simulink model "HANcoder_E407_TTA_Template_DS_V6"  (R2023a)
settings: Solver=FixedStepDiscrete  StartTime=0.0  StopTime=1  FixedStep=0.01  RelTol=1e-3
PreLoadFcn:
  | librarySetup
  | eval([bdroot,'_startup']) %Calling [modelName]_startup.m
values from neighbouring files (symbols this model uses):
  basic_cycle_duration_bc0 = TM_Reset_Board   + COMP_duration    (= 372)    [HANcoder_E407_TTA_Template_DS_V1_startup.m]    (also in HANcoder_E407_TTA_Template_DS_V2_startup.m; HANcoder_E407_TTA_Template_DS_V52_startup.m; HANcoder_E407_TTA_Template_DS_V5_startup.m; HANcoder_E407_TTA_Template_DS_V6_startup.m = 532)
  basic_cycle_duration_bc1 = basic_cycle_duration_bc0    (= 372)    [HANcoder_E407_TTA_Template_DS_V1_startup.m]    (also in HANcoder_E407_TTA_Template_DS_V2_startup.m; HANcoder_E407_TTA_Template_DS_V52_startup.m; HANcoder_E407_TTA_Template_DS_V5_startup.m; HANcoder_E407_TTA_Template_DS_V6_startup.m = 532)
  basic_cycle_duration_bc2 = basic_cycle_duration_bc0    (= 372)    [HANcoder_E407_TTA_Template_DS_V1_startup.m]    (also in HANcoder_E407_TTA_Template_DS_V2_startup.m; HANcoder_E407_TTA_Template_DS_V52_startup.m; HANcoder_E407_TTA_Template_DS_V5_startup.m; HANcoder_E407_TTA_Template_DS_V6_startup.m = 532)
  comm_delay_estimation1 = round(comm_delay_measured1*hardware_granularity/frequency_IRQ)    [HANcoder_E407_TTA_Template_DS_V1_startup.m]    (also in HANcoder_E407_TTA_Template_DS_V2_startup.m; HANcoder_E407_TTA_Template_DS_V52_startup.m; HANcoder_E407_TTA_Template_DS_V5_startup.m; HANcoder_E407_TTA_Template_DS_V6_startup.m)
  comm_delay_estimation2 = round(comm_delay_measured2*hardware_granularity/frequency_IRQ)    [HANcoder_E407_TTA_Template_DS_V1_startup.m]    (also in HANcoder_E407_TTA_Template_DS_V2_startup.m; HANcoder_E407_TTA_Template_DS_V52_startup.m; HANcoder_E407_TTA_Template_DS_V5_startup.m; HANcoder_E407_TTA_Template_DS_V6_startup.m)
  COMM_Period = 80    [HANcoder_E407_TTA_Template_DS_V1_startup.m]    (also in HANcoder_E407_TTA_Template_DS_V2_startup.m; HANcoder_E407_TTA_Template_DS_V52_startup.m; HANcoder_E407_TTA_Template_DS_V5_startup.m; HANcoder_E407_TTA_Template_DS_V6_startup.m = 120)
  COMM_Phase1 = Simulink.Parameter    [HANcoder_E407_TTA_Template_DS_V1_startup.m]    (also in HANcoder_E407_TTA_Template_DS_V2_startup.m; HANcoder_E407_TTA_Template_DS_V52_startup.m; HANcoder_E407_TTA_Template_DS_V5_startup.m; HANcoder_E407_TTA_Template_DS_V6_startup.m)
  COMM_Phase2 = Simulink.Parameter    [HANcoder_E407_TTA_Template_DS_V1_startup.m]    (also in HANcoder_E407_TTA_Template_DS_V2_startup.m; HANcoder_E407_TTA_Template_DS_V52_startup.m; HANcoder_E407_TTA_Template_DS_V5_startup.m; HANcoder_E407_TTA_Template_DS_V6_startup.m)
  COMM_Phase_init1 = Simulink.Parameter    [HANcoder_E407_TTA_Template_DS_V1_startup.m]    (also in HANcoder_E407_TTA_Template_DS_V2_startup.m; HANcoder_E407_TTA_Template_DS_V52_startup.m; HANcoder_E407_TTA_Template_DS_V5_startup.m; HANcoder_E407_TTA_Template_DS_V6_startup.m)
  COMM_Phase_init2 = Simulink.Parameter    [HANcoder_E407_TTA_Template_DS_V1_startup.m]    (also in HANcoder_E407_TTA_Template_DS_V2_startup.m; HANcoder_E407_TTA_Template_DS_V52_startup.m; HANcoder_E407_TTA_Template_DS_V5_startup.m; HANcoder_E407_TTA_Template_DS_V6_startup.m)
  COMP_duration = 4    [HANcoder_E407_TTA_Template_DS_V1_startup.m]    (also in HANcoder_E407_TTA_Template_DS_V2_startup.m; HANcoder_E407_TTA_Template_DS_V52_startup.m; HANcoder_E407_TTA_Template_DS_V5_startup.m; HANcoder_E407_TTA_Template_DS_V6_startup.m)
  frequency_IRQ = 100    [HANcoder_E407_TTA_Template_DS_V1_startup.m]    (also in HANcoder_E407_TTA_Template_DS_V2_startup.m; HANcoder_E407_TTA_Template_DS_V52_startup.m; HANcoder_E407_TTA_Template_DS_V5_startup.m; HANcoder_E407_TTA_Template_DS_V6_startup.m)
  idle_time_init = basic_cycle_duration_bc0 + basic_cycle_duration_bc1    (= 744)    [HANcoder_E407_TTA_Template_DS_V1_startup.m]    (also in HANcoder_E407_TTA_Template_DS_V2_startup.m; HANcoder_E407_TTA_Template_DS_V52_startup.m = 1116; HANcoder_E407_TTA_Template_DS_V5_startup.m = 1116; HANcoder_E407_TTA_Template_DS_V6_startup.m = 1596)
  L0b = 0.5    [HANcoder_E407_TTA_Template_DS_V52_startup.m]    (also in HANcoder_E407_TTA_Template_DS_V5_startup.m; HANcoder_E407_TTA_Template_DS_V6_startup.m)
  L0f = 5    [HANcoder_E407_TTA_Template_DS_V52_startup.m]    (also in HANcoder_E407_TTA_Template_DS_V5_startup.m; HANcoder_E407_TTA_Template_DS_V6_startup.m)
  L1f = 6    [HANcoder_E407_TTA_Template_DS_V52_startup.m]    (also in HANcoder_E407_TTA_Template_DS_V5_startup.m; HANcoder_E407_TTA_Template_DS_V6_startup.m)
  LA_Clock_Gr = 1    [HANcoder_E407_TTA_Template_DS_V1_startup.m]    (also in HANcoder_E407_TTA_Template_DS_V2_startup.m; HANcoder_E407_TTA_Template_DS_V52_startup.m; HANcoder_E407_TTA_Template_DS_V5_startup.m; HANcoder_E407_TTA_Template_DS_V6_startup.m)
  LA_COMM_dly = 1    [HANcoder_E407_TTA_Template_DS_V1_startup.m]    (also in HANcoder_E407_TTA_Template_DS_V2_startup.m; HANcoder_E407_TTA_Template_DS_V52_startup.m; HANcoder_E407_TTA_Template_DS_V5_startup.m; HANcoder_E407_TTA_Template_DS_V6_startup.m)
  LA_COMM_Err = 1    [HANcoder_E407_TTA_Template_DS_V1_startup.m]    (also in HANcoder_E407_TTA_Template_DS_V2_startup.m; HANcoder_E407_TTA_Template_DS_V52_startup.m; HANcoder_E407_TTA_Template_DS_V5_startup.m; HANcoder_E407_TTA_Template_DS_V6_startup.m)
  LA_E_Desync = 1    [HANcoder_E407_TTA_Template_DS_V1_startup.m]    (also in HANcoder_E407_TTA_Template_DS_V2_startup.m; HANcoder_E407_TTA_Template_DS_V52_startup.m; HANcoder_E407_TTA_Template_DS_V5_startup.m; HANcoder_E407_TTA_Template_DS_V6_startup.m)
  LA_MEX_Flag = 1    [HANcoder_E407_TTA_Template_DS_V1_startup.m]    (also in HANcoder_E407_TTA_Template_DS_V2_startup.m; HANcoder_E407_TTA_Template_DS_V52_startup.m; HANcoder_E407_TTA_Template_DS_V5_startup.m; HANcoder_E407_TTA_Template_DS_V6_startup.m)
  LA_Task_Act = 1    [HANcoder_E407_TTA_Template_DS_V1_startup.m]    (also in HANcoder_E407_TTA_Template_DS_V2_startup.m; HANcoder_E407_TTA_Template_DS_V52_startup.m; HANcoder_E407_TTA_Template_DS_V5_startup.m; HANcoder_E407_TTA_Template_DS_V6_startup.m)
  Master_Role = 1    [HANcoder_E407_TTA_Template_DS_V1_startup.m]    (also in HANcoder_E407_TTA_Template_DS_V2_startup.m; HANcoder_E407_TTA_Template_DS_V52_startup.m; HANcoder_E407_TTA_Template_DS_V5_startup.m; HANcoder_E407_TTA_Template_DS_V6_startup.m)
  matrix_rows = 3    [HANcoder_E407_TTA_Template_DS_V1_startup.m]    (also in HANcoder_E407_TTA_Template_DS_V2_startup.m; HANcoder_E407_TTA_Template_DS_V52_startup.m; HANcoder_E407_TTA_Template_DS_V5_startup.m; HANcoder_E407_TTA_Template_DS_V6_startup.m)
  max_desync = 15    [HANcoder_E407_TTA_Template_DS_V1_startup.m]    (also in HANcoder_E407_TTA_Template_DS_V2_startup.m; HANcoder_E407_TTA_Template_DS_V52_startup.m; HANcoder_E407_TTA_Template_DS_V5_startup.m; HANcoder_E407_TTA_Template_DS_V6_startup.m)
  max_num_msgs_CAN1 = 2^Tx_bit_number-1    (= 7)    [HANcoder_E407_TTA_Template_DS_V1_startup.m]    (also in HANcoder_E407_TTA_Template_DS_V2_startup.m; HANcoder_E407_TTA_Template_DS_V52_startup.m; HANcoder_E407_TTA_Template_DS_V5_startup.m; HANcoder_E407_TTA_Template_DS_V6_startup.m)
  max_num_msgs_CAN2 = max_num_msgs_CAN1    (= 7)    [HANcoder_E407_TTA_Template_DS_V1_startup.m]    (also in HANcoder_E407_TTA_Template_DS_V2_startup.m; HANcoder_E407_TTA_Template_DS_V52_startup.m; HANcoder_E407_TTA_Template_DS_V5_startup.m; HANcoder_E407_TTA_Template_DS_V6_startup.m)
  min_desync = (-1)*max_desync    (= -15)    [HANcoder_E407_TTA_Template_DS_V1_startup.m]    (also in HANcoder_E407_TTA_Template_DS_V2_startup.m; HANcoder_E407_TTA_Template_DS_V52_startup.m; HANcoder_E407_TTA_Template_DS_V5_startup.m; HANcoder_E407_TTA_Template_DS_V6_startup.m)
  PID_derivative = Simulink.Parameter    [HANcoder_E407_TTA_Template_DS_V52_startup.m]    (also in HANcoder_E407_TTA_Template_DS_V6_startup.m)
  PID_gain = Simulink.Parameter    [HANcoder_E407_TTA_Template_DS_V52_startup.m]    (also in HANcoder_E407_TTA_Template_DS_V6_startup.m)
  PID_integrator = Simulink.Parameter    [HANcoder_E407_TTA_Template_DS_V52_startup.m]    (also in HANcoder_E407_TTA_Template_DS_V6_startup.m)
  PotValue1_ID = 22    [HANcoder_E407_TTA_Template_DS_V1_startup.m]    (also in HANcoder_E407_TTA_Template_DS_V2_startup.m; HANcoder_E407_TTA_Template_DS_V52_startup.m; HANcoder_E407_TTA_Template_DS_V5_startup.m; HANcoder_E407_TTA_Template_DS_V6_startup.m)
  PotValue2_ID = 23    [HANcoder_E407_TTA_Template_DS_V1_startup.m]    (also in HANcoder_E407_TTA_Template_DS_V2_startup.m; HANcoder_E407_TTA_Template_DS_V52_startup.m; HANcoder_E407_TTA_Template_DS_V5_startup.m; HANcoder_E407_TTA_Template_DS_V6_startup.m)
  PotValue3_ID = 24    [HANcoder_E407_TTA_Template_DS_V1_startup.m]    (also in HANcoder_E407_TTA_Template_DS_V2_startup.m; HANcoder_E407_TTA_Template_DS_V52_startup.m; HANcoder_E407_TTA_Template_DS_V5_startup.m; HANcoder_E407_TTA_Template_DS_V6_startup.m)
  script_run = Simulink.Parameter    [HANcoder_E407_TTA_Template_DS_V1_startup.m]    (also in HANcoder_E407_TTA_Template_DS_V2_startup.m; HANcoder_E407_TTA_Template_DS_V52_startup.m; HANcoder_E407_TTA_Template_DS_V5_startup.m; HANcoder_E407_TTA_Template_DS_V6_startup.m)
  Slave_Role = 2    [HANcoder_E407_TTA_Template_DS_V1_startup.m]    (also in HANcoder_E407_TTA_Template_DS_V2_startup.m; HANcoder_E407_TTA_Template_DS_V52_startup.m; HANcoder_E407_TTA_Template_DS_V5_startup.m; HANcoder_E407_TTA_Template_DS_V6_startup.m)
  Sync_ID = 1    [HANcoder_E407_TTA_Template_DS_V1_startup.m]    (also in HANcoder_E407_TTA_Template_DS_V2_startup.m; HANcoder_E407_TTA_Template_DS_V52_startup.m; HANcoder_E407_TTA_Template_DS_V5_startup.m; HANcoder_E407_TTA_Template_DS_V6_startup.m)
  TM_Check_PotValue1 = TM_COMM_PotValue1 + COMM_duration    (= 174)    [HANcoder_E407_TTA_Template_DS_V1_startup.m]    (also in HANcoder_E407_TTA_Template_DS_V2_startup.m; HANcoder_E407_TTA_Template_DS_V52_startup.m; HANcoder_E407_TTA_Template_DS_V5_startup.m; HANcoder_E407_TTA_Template_DS_V6_startup.m = 254)
  TM_Check_PotValue2 = TM_COMM_PotValue2 + COMM_duration    (= 258)    [HANcoder_E407_TTA_Template_DS_V1_startup.m]    (also in HANcoder_E407_TTA_Template_DS_V2_startup.m; HANcoder_E407_TTA_Template_DS_V52_startup.m; HANcoder_E407_TTA_Template_DS_V5_startup.m; HANcoder_E407_TTA_Template_DS_V6_startup.m = 378)
  TM_Check_PotValue3 = TM_COMM_PotValue3 + COMM_duration    (= 342)    [HANcoder_E407_TTA_Template_DS_V1_startup.m]    (also in HANcoder_E407_TTA_Template_DS_V2_startup.m; HANcoder_E407_TTA_Template_DS_V52_startup.m; HANcoder_E407_TTA_Template_DS_V5_startup.m; HANcoder_E407_TTA_Template_DS_V6_startup.m = 502)
  TM_Check_Sync = TM_COMM_Sync   + COMM_duration    (= 80)    [HANcoder_E407_TTA_Template_DS_V1_startup.m]    (also in HANcoder_E407_TTA_Template_DS_V2_startup.m; HANcoder_E407_TTA_Template_DS_V52_startup.m; HANcoder_E407_TTA_Template_DS_V5_startup.m; HANcoder_E407_TTA_Template_DS_V6_startup.m = 120)
  TM_Check_TOuts = TM_Count_Vote3 + COMP_duration    (= 356)    [HANcoder_E407_TTA_Template_DS_V1_startup.m]    (also in HANcoder_E407_TTA_Template_DS_V2_startup.m; HANcoder_E407_TTA_Template_DS_V52_startup.m; HANcoder_E407_TTA_Template_DS_V5_startup.m; HANcoder_E407_TTA_Template_DS_V6_startup.m = 516)
  TM_Check_Trailer1Articulation = TM_COMM_Trailer1Articulation + COMM_duration    (= 170)    [HANcoder_E407_TTA_Template_DS_V1_startup.m]    (also in HANcoder_E407_TTA_Template_DS_V2_startup.m; HANcoder_E407_TTA_Template_DS_V52_startup.m; HANcoder_E407_TTA_Template_DS_V5_startup.m; HANcoder_E407_TTA_Template_DS_V6_startup.m = 250)
  TM_Check_Trailer2Articulation = TM_COMM_Trailer2Articulation + COMM_duration    (= 254)    [HANcoder_E407_TTA_Template_DS_V1_startup.m]    (also in HANcoder_E407_TTA_Template_DS_V2_startup.m; HANcoder_E407_TTA_Template_DS_V52_startup.m; HANcoder_E407_TTA_Template_DS_V5_startup.m; HANcoder_E407_TTA_Template_DS_V6_startup.m = 374)
  TM_Check_Vote1 = TM_COMM_Vote1  + COMM_duration    (= 172)    [HANcoder_E407_TTA_Template_DS_V1_startup.m]    (also in HANcoder_E407_TTA_Template_DS_V2_startup.m; HANcoder_E407_TTA_Template_DS_V52_startup.m; HANcoder_E407_TTA_Template_DS_V5_startup.m; HANcoder_E407_TTA_Template_DS_V6_startup.m = 252)
  TM_Check_Vote2 = TM_COMM_Vote2  + COMM_duration    (= 260)    [HANcoder_E407_TTA_Template_DS_V1_startup.m]    (also in HANcoder_E407_TTA_Template_DS_V2_startup.m; HANcoder_E407_TTA_Template_DS_V52_startup.m; HANcoder_E407_TTA_Template_DS_V5_startup.m; HANcoder_E407_TTA_Template_DS_V6_startup.m = 380)
  TM_Check_Vote3 = TM_COMM_Vote3  + COMM_duration    (= 348)    [HANcoder_E407_TTA_Template_DS_V1_startup.m]    (also in HANcoder_E407_TTA_Template_DS_V2_startup.m; HANcoder_E407_TTA_Template_DS_V52_startup.m; HANcoder_E407_TTA_Template_DS_V5_startup.m; HANcoder_E407_TTA_Template_DS_V6_startup.m = 508)
  TM_COMM_PotValue1 = TM_ReadPot + COMP_duration    (= 94)    [HANcoder_E407_TTA_Template_DS_V1_startup.m]    (also in HANcoder_E407_TTA_Template_DS_V2_startup.m; HANcoder_E407_TTA_Template_DS_V52_startup.m; HANcoder_E407_TTA_Template_DS_V5_startup.m; HANcoder_E407_TTA_Template_DS_V6_startup.m = 134)
  TM_COMM_PotValue2 = TM_Check_PotValue1 + COMP_duration    (= 178)    [HANcoder_E407_TTA_Template_DS_V1_startup.m]    (also in HANcoder_E407_TTA_Template_DS_V2_startup.m; HANcoder_E407_TTA_Template_DS_V52_startup.m; HANcoder_E407_TTA_Template_DS_V5_startup.m; HANcoder_E407_TTA_Template_DS_V6_startup.m = 258)
  TM_COMM_PotValue3 = TM_Check_PotValue2 + COMP_duration    (= 262)    [HANcoder_E407_TTA_Template_DS_V1_startup.m]    (also in HANcoder_E407_TTA_Template_DS_V2_startup.m; HANcoder_E407_TTA_Template_DS_V52_startup.m; HANcoder_E407_TTA_Template_DS_V5_startup.m; HANcoder_E407_TTA_Template_DS_V6_startup.m = 382)
  TM_COMM_Sync = basic_cycle_start    (= 0)    [HANcoder_E407_TTA_Template_DS_V1_startup.m]    (also in HANcoder_E407_TTA_Template_DS_V2_startup.m; HANcoder_E407_TTA_Template_DS_V52_startup.m; HANcoder_E407_TTA_Template_DS_V5_startup.m; HANcoder_E407_TTA_Template_DS_V6_startup.m)
  TM_COMM_Trailer1Articulation = TM_Update_LT_2 + COMP_duration    (= 90)    [HANcoder_E407_TTA_Template_DS_V1_startup.m]    (also in HANcoder_E407_TTA_Template_DS_V2_startup.m; HANcoder_E407_TTA_Template_DS_V52_startup.m; HANcoder_E407_TTA_Template_DS_V5_startup.m; HANcoder_E407_TTA_Template_DS_V6_startup.m = 130)
  TM_COMM_Trailer2Articulation = TM_Check_Trailer1Articulation + COMP_duration    (= 174)    [HANcoder_E407_TTA_Template_DS_V1_startup.m]    (also in HANcoder_E407_TTA_Template_DS_V2_startup.m; HANcoder_E407_TTA_Template_DS_V52_startup.m; HANcoder_E407_TTA_Template_DS_V5_startup.m; HANcoder_E407_TTA_Template_DS_V6_startup.m = 254)
  TM_COMM_Vote1 = TM_Vote_Dec    + COMP_duration    (= 92)    [HANcoder_E407_TTA_Template_DS_V1_startup.m]    (also in HANcoder_E407_TTA_Template_DS_V2_startup.m; HANcoder_E407_TTA_Template_DS_V52_startup.m; HANcoder_E407_TTA_Template_DS_V5_startup.m; HANcoder_E407_TTA_Template_DS_V6_startup.m = 132)
  TM_COMM_Vote2 = TM_Count_Vote1 + COMP_duration    (= 180)    [HANcoder_E407_TTA_Template_DS_V1_startup.m]    (also in HANcoder_E407_TTA_Template_DS_V2_startup.m; HANcoder_E407_TTA_Template_DS_V52_startup.m; HANcoder_E407_TTA_Template_DS_V5_startup.m; HANcoder_E407_TTA_Template_DS_V6_startup.m = 260)
  TM_COMM_Vote3 = TM_Count_Vote2 + COMP_duration    (= 268)    [HANcoder_E407_TTA_Template_DS_V1_startup.m]    (also in HANcoder_E407_TTA_Template_DS_V2_startup.m; HANcoder_E407_TTA_Template_DS_V52_startup.m; HANcoder_E407_TTA_Template_DS_V5_startup.m; HANcoder_E407_TTA_Template_DS_V6_startup.m = 388)
  TM_Count_Vote1 = TM_Check_Vote1 + COMP_duration    (= 176)    [HANcoder_E407_TTA_Template_DS_V1_startup.m]    (also in HANcoder_E407_TTA_Template_DS_V2_startup.m; HANcoder_E407_TTA_Template_DS_V52_startup.m; HANcoder_E407_TTA_Template_DS_V5_startup.m; HANcoder_E407_TTA_Template_DS_V6_startup.m = 256)
  TM_Count_Vote2 = TM_Check_Vote2 + COMP_duration    (= 264)    [HANcoder_E407_TTA_Template_DS_V1_startup.m]    (also in HANcoder_E407_TTA_Template_DS_V2_startup.m; HANcoder_E407_TTA_Template_DS_V52_startup.m; HANcoder_E407_TTA_Template_DS_V5_startup.m; HANcoder_E407_TTA_Template_DS_V6_startup.m = 384)
  TM_Count_Vote3 = TM_Check_Vote3 + COMP_duration    (= 352)    [HANcoder_E407_TTA_Template_DS_V1_startup.m]    (also in HANcoder_E407_TTA_Template_DS_V2_startup.m; HANcoder_E407_TTA_Template_DS_V52_startup.m; HANcoder_E407_TTA_Template_DS_V5_startup.m; HANcoder_E407_TTA_Template_DS_V6_startup.m = 512)
  TM_Data_bc0 = TM_COMM_Sync    (= 0)    [HANcoder_E407_TTA_Template_DS_V1_startup.m]    (also in HANcoder_E407_TTA_Template_DS_V2_startup.m; HANcoder_E407_TTA_Template_DS_V52_startup.m; HANcoder_E407_TTA_Template_DS_V5_startup.m; HANcoder_E407_TTA_Template_DS_V6_startup.m)
  TM_Data_bc1 = TM_Data_bc0(1:4)    [HANcoder_E407_TTA_Template_DS_V1_startup.m]    (also in HANcoder_E407_TTA_Template_DS_V2_startup.m; HANcoder_E407_TTA_Template_DS_V52_startup.m; HANcoder_E407_TTA_Template_DS_V5_startup.m; HANcoder_E407_TTA_Template_DS_V6_startup.m)
  TM_Data_bc2 = TM_Data_bc0(1:4)    [HANcoder_E407_TTA_Template_DS_V1_startup.m]    (also in HANcoder_E407_TTA_Template_DS_V2_startup.m; HANcoder_E407_TTA_Template_DS_V52_startup.m; HANcoder_E407_TTA_Template_DS_V5_startup.m; HANcoder_E407_TTA_Template_DS_V6_startup.m)
  TM_InverseKinematics = TM_Check_Trailer2Articulation + COMP_duration    (= 258)    [HANcoder_E407_TTA_Template_DS_V1_startup.m]    (also in HANcoder_E407_TTA_Template_DS_V2_startup.m; HANcoder_E407_TTA_Template_DS_V52_startup.m; HANcoder_E407_TTA_Template_DS_V5_startup.m; HANcoder_E407_TTA_Template_DS_V6_startup.m = 378)
  TM_New_Master = TM_Check_TOuts + COMP_duration    (= 360)    [HANcoder_E407_TTA_Template_DS_V1_startup.m]    (also in HANcoder_E407_TTA_Template_DS_V2_startup.m; HANcoder_E407_TTA_Template_DS_V52_startup.m; HANcoder_E407_TTA_Template_DS_V5_startup.m; HANcoder_E407_TTA_Template_DS_V6_startup.m = 520)
  TM_PotVote = TM_COMM_PotValue3 + COMP_duration    (= 266)    [HANcoder_E407_TTA_Template_DS_V1_startup.m]    (also in HANcoder_E407_TTA_Template_DS_V2_startup.m; HANcoder_E407_TTA_Template_DS_V52_startup.m; HANcoder_E407_TTA_Template_DS_V5_startup.m; HANcoder_E407_TTA_Template_DS_V6_startup.m = 386)
  TM_ReadPot = TM_Update_LT_2 + COMP_duration    (= 90)    [HANcoder_E407_TTA_Template_DS_V1_startup.m]    (also in HANcoder_E407_TTA_Template_DS_V2_startup.m; HANcoder_E407_TTA_Template_DS_V52_startup.m; HANcoder_E407_TTA_Template_DS_V5_startup.m; HANcoder_E407_TTA_Template_DS_V6_startup.m = 130)
  TM_Reset_Board = TM_Reset_Var   + COMP_duration    (= 368)    [HANcoder_E407_TTA_Template_DS_V1_startup.m]    (also in HANcoder_E407_TTA_Template_DS_V2_startup.m; HANcoder_E407_TTA_Template_DS_V52_startup.m; HANcoder_E407_TTA_Template_DS_V5_startup.m; HANcoder_E407_TTA_Template_DS_V6_startup.m = 528)
  TM_Reset_Var = TM_New_Master  + COMP_duration    (= 364)    [HANcoder_E407_TTA_Template_DS_V1_startup.m]    (also in HANcoder_E407_TTA_Template_DS_V2_startup.m; HANcoder_E407_TTA_Template_DS_V52_startup.m; HANcoder_E407_TTA_Template_DS_V5_startup.m; HANcoder_E407_TTA_Template_DS_V6_startup.m = 524)
  TM_Reset_Var_bc1 = TM_Data_bc1(end) + COMP_duration    [HANcoder_E407_TTA_Template_DS_V1_startup.m]    (also in HANcoder_E407_TTA_Template_DS_V2_startup.m; HANcoder_E407_TTA_Template_DS_V52_startup.m; HANcoder_E407_TTA_Template_DS_V5_startup.m; HANcoder_E407_TTA_Template_DS_V6_startup.m)
  TM_Reset_Var_bc1_2 = TM_Reset_Var_bc1 +2    [HANcoder_E407_TTA_Template_DS_V1_startup.m]    (also in HANcoder_E407_TTA_Template_DS_V2_startup.m; HANcoder_E407_TTA_Template_DS_V52_startup.m; HANcoder_E407_TTA_Template_DS_V5_startup.m; HANcoder_E407_TTA_Template_DS_V6_startup.m)
  TM_Reset_Var_bc2 = TM_Data_bc2(end) + COMP_duration    [HANcoder_E407_TTA_Template_DS_V1_startup.m]    (also in HANcoder_E407_TTA_Template_DS_V2_startup.m; HANcoder_E407_TTA_Template_DS_V52_startup.m; HANcoder_E407_TTA_Template_DS_V5_startup.m; HANcoder_E407_TTA_Template_DS_V6_startup.m)
  TM_Reset_Var_bc2_2 = TM_Reset_Var_bc2 +2    [HANcoder_E407_TTA_Template_DS_V1_startup.m]    (also in HANcoder_E407_TTA_Template_DS_V2_startup.m; HANcoder_E407_TTA_Template_DS_V52_startup.m; HANcoder_E407_TTA_Template_DS_V5_startup.m; HANcoder_E407_TTA_Template_DS_V6_startup.m)
  TM_Type_bc0 = COMM    (= 0)    [HANcoder_E407_TTA_Template_DS_V1_startup.m]    (also in HANcoder_E407_TTA_Template_DS_V2_startup.m; HANcoder_E407_TTA_Template_DS_V52_startup.m; HANcoder_E407_TTA_Template_DS_V5_startup.m; HANcoder_E407_TTA_Template_DS_V6_startup.m)
  TM_Type_bc1 = TM_Type_bc0(1:4)    [HANcoder_E407_TTA_Template_DS_V1_startup.m]    (also in HANcoder_E407_TTA_Template_DS_V2_startup.m; HANcoder_E407_TTA_Template_DS_V52_startup.m; HANcoder_E407_TTA_Template_DS_V5_startup.m; HANcoder_E407_TTA_Template_DS_V6_startup.m)
  TM_Type_bc2 = TM_Type_bc0(1:4)    [HANcoder_E407_TTA_Template_DS_V1_startup.m]    (also in HANcoder_E407_TTA_Template_DS_V2_startup.m; HANcoder_E407_TTA_Template_DS_V52_startup.m; HANcoder_E407_TTA_Template_DS_V5_startup.m; HANcoder_E407_TTA_Template_DS_V6_startup.m)
  TM_Update_LT = TM_Check_Sync  + COMP_duration    (= 84)    [HANcoder_E407_TTA_Template_DS_V1_startup.m]    (also in HANcoder_E407_TTA_Template_DS_V2_startup.m; HANcoder_E407_TTA_Template_DS_V52_startup.m; HANcoder_E407_TTA_Template_DS_V5_startup.m; HANcoder_E407_TTA_Template_DS_V6_startup.m = 124)
  TM_Update_LT_2 = TM_Update_LT   + 2    (= 86)    [HANcoder_E407_TTA_Template_DS_V1_startup.m]    (also in HANcoder_E407_TTA_Template_DS_V2_startup.m; HANcoder_E407_TTA_Template_DS_V52_startup.m; HANcoder_E407_TTA_Template_DS_V5_startup.m; HANcoder_E407_TTA_Template_DS_V6_startup.m = 126)
  TM_Vote_Dec = TM_Update_LT   + COMP_duration    (= 88)    [HANcoder_E407_TTA_Template_DS_V1_startup.m]    (also in HANcoder_E407_TTA_Template_DS_V2_startup.m; HANcoder_E407_TTA_Template_DS_V52_startup.m; HANcoder_E407_TTA_Template_DS_V5_startup.m; HANcoder_E407_TTA_Template_DS_V6_startup.m = 128)
  Tractor_Board1 = 11    [HANcoder_E407_TTA_Template_DS_V1_startup.m]    (also in HANcoder_E407_TTA_Template_DS_V2_startup.m = 1; HANcoder_E407_TTA_Template_DS_V52_startup.m = 1; HANcoder_E407_TTA_Template_DS_V5_startup.m = 1; HANcoder_E407_TTA_Template_DS_V6_startup.m = 1)
  Tractor_Board2 = 12    [HANcoder_E407_TTA_Template_DS_V1_startup.m]    (also in HANcoder_E407_TTA_Template_DS_V2_startup.m = 2; HANcoder_E407_TTA_Template_DS_V52_startup.m = 2; HANcoder_E407_TTA_Template_DS_V5_startup.m = 2; HANcoder_E407_TTA_Template_DS_V6_startup.m = 2)
  Tractor_Board3 = 13    [HANcoder_E407_TTA_Template_DS_V1_startup.m]    (also in HANcoder_E407_TTA_Template_DS_V2_startup.m = 3; HANcoder_E407_TTA_Template_DS_V52_startup.m = 3; HANcoder_E407_TTA_Template_DS_V5_startup.m = 3; HANcoder_E407_TTA_Template_DS_V6_startup.m = 3)
  Trailer1_Articulation_ID = 31    [HANcoder_E407_TTA_Template_DS_V1_startup.m]    (also in HANcoder_E407_TTA_Template_DS_V2_startup.m; HANcoder_E407_TTA_Template_DS_V52_startup.m; HANcoder_E407_TTA_Template_DS_V5_startup.m; HANcoder_E407_TTA_Template_DS_V6_startup.m)
  Trailer1_Board1 = 2    [HANcoder_E407_TTA_Template_DS_V1_startup.m]    (also in HANcoder_E407_TTA_Template_DS_V2_startup.m = 4; HANcoder_E407_TTA_Template_DS_V52_startup.m = 4; HANcoder_E407_TTA_Template_DS_V5_startup.m = 4; HANcoder_E407_TTA_Template_DS_V6_startup.m = 4)
  Trailer1_Board2 = 3    [HANcoder_E407_TTA_Template_DS_V1_startup.m]    (also in HANcoder_E407_TTA_Template_DS_V2_startup.m = 5; HANcoder_E407_TTA_Template_DS_V52_startup.m = 5; HANcoder_E407_TTA_Template_DS_V5_startup.m = 5; HANcoder_E407_TTA_Template_DS_V6_startup.m = 5)
  Trailer1_Board3 = 4    [HANcoder_E407_TTA_Template_DS_V1_startup.m]    (also in HANcoder_E407_TTA_Template_DS_V2_startup.m = 6; HANcoder_E407_TTA_Template_DS_V52_startup.m = 6; HANcoder_E407_TTA_Template_DS_V5_startup.m = 6; HANcoder_E407_TTA_Template_DS_V6_startup.m = 6)
  Trailer2_Articulation_ID = 32    [HANcoder_E407_TTA_Template_DS_V1_startup.m]    (also in HANcoder_E407_TTA_Template_DS_V2_startup.m; HANcoder_E407_TTA_Template_DS_V52_startup.m; HANcoder_E407_TTA_Template_DS_V5_startup.m; HANcoder_E407_TTA_Template_DS_V6_startup.m)
  Trailer2_Board1 = 5    [HANcoder_E407_TTA_Template_DS_V1_startup.m]    (also in HANcoder_E407_TTA_Template_DS_V2_startup.m = 7; HANcoder_E407_TTA_Template_DS_V52_startup.m = 7; HANcoder_E407_TTA_Template_DS_V5_startup.m = 7; HANcoder_E407_TTA_Template_DS_V6_startup.m = 7)
  Trailer2_Board2 = 6    [HANcoder_E407_TTA_Template_DS_V1_startup.m]    (also in HANcoder_E407_TTA_Template_DS_V2_startup.m = 8; HANcoder_E407_TTA_Template_DS_V52_startup.m = 8; HANcoder_E407_TTA_Template_DS_V5_startup.m = 8; HANcoder_E407_TTA_Template_DS_V6_startup.m = 8)
  Trailer2_Board3 = 7    [HANcoder_E407_TTA_Template_DS_V1_startup.m]    (also in HANcoder_E407_TTA_Template_DS_V2_startup.m = 9; HANcoder_E407_TTA_Template_DS_V52_startup.m = 9; HANcoder_E407_TTA_Template_DS_V5_startup.m = 9; HANcoder_E407_TTA_Template_DS_V6_startup.m = 9)
  V1 = -0.000000001    (= -1e-09)    [HANcoder_E407_TTA_Template_DS_V52_startup.m]    (also in HANcoder_E407_TTA_Template_DS_V5_startup.m; HANcoder_E407_TTA_Template_DS_V6_startup.m)
  V2 = -0.000000001    (= -1e-09)    [HANcoder_E407_TTA_Template_DS_V52_startup.m]    (also in HANcoder_E407_TTA_Template_DS_V5_startup.m; HANcoder_E407_TTA_Template_DS_V6_startup.m)
  Vote1_ID = 11    [HANcoder_E407_TTA_Template_DS_V1_startup.m]    (also in HANcoder_E407_TTA_Template_DS_V2_startup.m; HANcoder_E407_TTA_Template_DS_V52_startup.m; HANcoder_E407_TTA_Template_DS_V5_startup.m; HANcoder_E407_TTA_Template_DS_V6_startup.m)
  Vote2_ID = 12    [HANcoder_E407_TTA_Template_DS_V1_startup.m]    (also in HANcoder_E407_TTA_Template_DS_V2_startup.m; HANcoder_E407_TTA_Template_DS_V52_startup.m; HANcoder_E407_TTA_Template_DS_V5_startup.m; HANcoder_E407_TTA_Template_DS_V6_startup.m)
  Vote3_ID = 13    [HANcoder_E407_TTA_Template_DS_V1_startup.m]    (also in HANcoder_E407_TTA_Template_DS_V2_startup.m; HANcoder_E407_TTA_Template_DS_V52_startup.m; HANcoder_E407_TTA_Template_DS_V5_startup.m; HANcoder_E407_TTA_Template_DS_V6_startup.m)
undefined symbols (not defined in the file or in its folder): A0, A1, A2, A3, A4, A5, CON2, CON3, CON4, D10, D12, D13, D6, D7, D8, D9
libraries: hdlsllib x136, simulink x39, HANcoder_STM32_Target x31, simulink_extras x8, dspstat3 x2, slpidlib x1
(part 14 of 42)

== system HANcoder_E407_TTA_Template_DS_V6/HANcoder STM32 Target - E407-STM32 algorithm/TTA CAN System/CAN2 Recieve1/RxID_CAN/PotValue2_ID_CAN3/CAN receive1 ==
  In1 : Inport
  Enabled Subsystem : Subsystem  TreatAsAtomicUnit=on
  S-Function : M-S-Function  FunctionName=sfcn_can_receive  Parameters=tsamp, canBus, outputNumber, dataType, byteOrder
  Out1 : Outport  VectorParamsAs1DForOutWhenUnconnected=off
  Out2 : Outport  Port=2  VectorParamsAs1DForOutWhenUnconnected=off
  Out3 : Outport  Port=3  VectorParamsAs1DForOutWhenUnconnected=off
  Out4 : Outport  Port=4  VectorParamsAs1DForOutWhenUnconnected=off
  Out5 : Outport  Port=5  VectorParamsAs1DForOutWhenUnconnected=off
  Out6 : Outport  Port=6  VectorParamsAs1DForOutWhenUnconnected=off
  Out7 : Outport  Port=7  VectorParamsAs1DForOutWhenUnconnected=off
  Out8 : Outport  Port=8  VectorParamsAs1DForOutWhenUnconnected=off
  Out9 : Outport  Port=9  VectorParamsAs1DForOutWhenUnconnected=off
  wires:
  In1/1 -> S-Function/1
  S-Function/1 -> Enabled Subsystem/Enable, Out1/1
  S-Function/2 -> Enabled Subsystem/1(In1)
  S-Function/3 -> Enabled Subsystem/2(In2)
  Enabled Subsystem/1(Out1) -> Out2/1
  Enabled Subsystem/2(Out2) -> Out3/1
  Enabled Subsystem/3(Out3) -> Out4/1
  Enabled Subsystem/4(Out4) -> Out5/1
  Enabled Subsystem/5(Out5) -> Out6/1
  Enabled Subsystem/6(Out6) -> Out7/1
  Enabled Subsystem/7(Out7) -> Out8/1
  Enabled Subsystem/8(Out8) -> Out9/1
  S-Function/6 -> Enabled Subsystem/5(In5)
  S-Function/7 -> Enabled Subsystem/6(In6)
  S-Function/8 -> Enabled Subsystem/7(In7)
  S-Function/5 -> Enabled Subsystem/4(In4)
  S-Function/4 -> Enabled Subsystem/3(In3)
  S-Function/9 -> Enabled Subsystem/8(In8)

== system HANcoder_E407_TTA_Template_DS_V6/HANcoder STM32 Target - E407-STM32 algorithm/TTA CAN System/CAN2 Recieve1/RxID_CAN/PotValue2_ID_CAN4/CAN receive1 ==
  In1 : Inport
  Enabled Subsystem : Subsystem  TreatAsAtomicUnit=on
  S-Function : M-S-Function  FunctionName=sfcn_can_receive  Parameters=tsamp, canBus, outputNumber, dataType, byteOrder
  Out1 : Outport  VectorParamsAs1DForOutWhenUnconnected=off
  Out2 : Outport  Port=2  VectorParamsAs1DForOutWhenUnconnected=off
  Out3 : Outport  Port=3  VectorParamsAs1DForOutWhenUnconnected=off
  Out4 : Outport  Port=4  VectorParamsAs1DForOutWhenUnconnected=off
  Out5 : Outport  Port=5  VectorParamsAs1DForOutWhenUnconnected=off
  Out6 : Outport  Port=6  VectorParamsAs1DForOutWhenUnconnected=off
  Out7 : Outport  Port=7  VectorParamsAs1DForOutWhenUnconnected=off
  Out8 : Outport  Port=8  VectorParamsAs1DForOutWhenUnconnected=off
  Out9 : Outport  Port=9  VectorParamsAs1DForOutWhenUnconnected=off
  wires:
  In1/1 -> S-Function/1
  S-Function/1 -> Enabled Subsystem/Enable, Out1/1
  S-Function/2 -> Enabled Subsystem/1(In1)
  S-Function/3 -> Enabled Subsystem/2(In2)
  Enabled Subsystem/1(Out1) -> Out2/1
  Enabled Subsystem/2(Out2) -> Out3/1
  Enabled Subsystem/3(Out3) -> Out4/1
  Enabled Subsystem/4(Out4) -> Out5/1
  Enabled Subsystem/5(Out5) -> Out6/1
  Enabled Subsystem/6(Out6) -> Out7/1
  Enabled Subsystem/7(Out7) -> Out8/1
  Enabled Subsystem/8(Out8) -> Out9/1
  S-Function/6 -> Enabled Subsystem/5(In5)
  S-Function/7 -> Enabled Subsystem/6(In6)
  S-Function/8 -> Enabled Subsystem/7(In7)
  S-Function/5 -> Enabled Subsystem/4(In4)
  S-Function/4 -> Enabled Subsystem/3(In3)
  S-Function/9 -> Enabled Subsystem/8(In8)

== system HANcoder_E407_TTA_Template_DS_V6/HANcoder STM32 Target - E407-STM32 algorithm/TTA CAN System/CAN2 Recieve1/RxID_CAN/PotValue2_ID_CAN5/CAN receive1 ==
  In1 : Inport
  Enabled Subsystem : Subsystem  TreatAsAtomicUnit=on
  S-Function : M-S-Function  FunctionName=sfcn_can_receive  Parameters=tsamp, canBus, outputNumber, dataType, byteOrder
  Out1 : Outport  VectorParamsAs1DForOutWhenUnconnected=off
  Out2 : Outport  Port=2  VectorParamsAs1DForOutWhenUnconnected=off
  Out3 : Outport  Port=3  VectorParamsAs1DForOutWhenUnconnected=off
  Out4 : Outport  Port=4  VectorParamsAs1DForOutWhenUnconnected=off
  Out5 : Outport  Port=5  VectorParamsAs1DForOutWhenUnconnected=off
  Out6 : Outport  Port=6  VectorParamsAs1DForOutWhenUnconnected=off
  Out7 : Outport  Port=7  VectorParamsAs1DForOutWhenUnconnected=off
  Out8 : Outport  Port=8  VectorParamsAs1DForOutWhenUnconnected=off
  Out9 : Outport  Port=9  VectorParamsAs1DForOutWhenUnconnected=off
  wires:
  In1/1 -> S-Function/1
  S-Function/1 -> Enabled Subsystem/Enable, Out1/1
  S-Function/2 -> Enabled Subsystem/1(In1)
  S-Function/3 -> Enabled Subsystem/2(In2)
  Enabled Subsystem/1(Out1) -> Out2/1
  Enabled Subsystem/2(Out2) -> Out3/1
  Enabled Subsystem/3(Out3) -> Out4/1
  Enabled Subsystem/4(Out4) -> Out5/1
  Enabled Subsystem/5(Out5) -> Out6/1
  Enabled Subsystem/6(Out6) -> Out7/1
  Enabled Subsystem/7(Out7) -> Out8/1
  Enabled Subsystem/8(Out8) -> Out9/1
  S-Function/6 -> Enabled Subsystem/5(In5)
  S-Function/7 -> Enabled Subsystem/6(In6)
  S-Function/8 -> Enabled Subsystem/7(In7)
  S-Function/5 -> Enabled Subsystem/4(In4)
  S-Function/4 -> Enabled Subsystem/3(In3)
  S-Function/9 -> Enabled Subsystem/8(In8)

== system HANcoder_E407_TTA_Template_DS_V6/HANcoder STM32 Target - E407-STM32 algorithm/TTA CAN System/CAN2 Recieve1/RxID_CAN/PotValue2_ID_CAN6/CAN receive1 ==
  In1 : Inport
  Enabled Subsystem : Subsystem  TreatAsAtomicUnit=on
  S-Function : M-S-Function  FunctionName=sfcn_can_receive  Parameters=tsamp, canBus, outputNumber, dataType, byteOrder
  Out1 : Outport  VectorParamsAs1DForOutWhenUnconnected=off
  Out2 : Outport  Port=2  VectorParamsAs1DForOutWhenUnconnected=off
  Out3 : Outport  Port=3  VectorParamsAs1DForOutWhenUnconnected=off
  Out4 : Outport  Port=4  VectorParamsAs1DForOutWhenUnconnected=off
  Out5 : Outport  Port=5  VectorParamsAs1DForOutWhenUnconnected=off
  Out6 : Outport  Port=6  VectorParamsAs1DForOutWhenUnconnected=off
  Out7 : Outport  Port=7  VectorParamsAs1DForOutWhenUnconnected=off
  Out8 : Outport  Port=8  VectorParamsAs1DForOutWhenUnconnected=off
  Out9 : Outport  Port=9  VectorParamsAs1DForOutWhenUnconnected=off
  wires:
  In1/1 -> S-Function/1
  S-Function/1 -> Enabled Subsystem/Enable, Out1/1
  S-Function/2 -> Enabled Subsystem/1(In1)
  S-Function/3 -> Enabled Subsystem/2(In2)
  Enabled Subsystem/1(Out1) -> Out2/1
  Enabled Subsystem/2(Out2) -> Out3/1
  Enabled Subsystem/3(Out3) -> Out4/1
  Enabled Subsystem/4(Out4) -> Out5/1
  Enabled Subsystem/5(Out5) -> Out6/1
  Enabled Subsystem/6(Out6) -> Out7/1
  Enabled Subsystem/7(Out7) -> Out8/1
  Enabled Subsystem/8(Out8) -> Out9/1
  S-Function/6 -> Enabled Subsystem/5(In5)
  S-Function/7 -> Enabled Subsystem/6(In6)
  S-Function/8 -> Enabled Subsystem/7(In7)
  S-Function/5 -> Enabled Subsystem/4(In4)
  S-Function/4 -> Enabled Subsystem/3(In3)
  S-Function/9 -> Enabled Subsystem/8(In8)

== system HANcoder_E407_TTA_Template_DS_V6/HANcoder STM32 Target - E407-STM32 algorithm/TTA CAN System/CAN2 Recieve1/RxID_CAN/Sync_ID_CAN/CAN receive1 ==
  In1 : Inport
  Enabled Subsystem : Subsystem  TreatAsAtomicUnit=on
  S-Function : M-S-Function  FunctionName=sfcn_can_receive  Parameters=tsamp, canBus, outputNumber, dataType, byteOrder
  Out1 : Outport  VectorParamsAs1DForOutWhenUnconnected=off
  Out2 : Outport  Port=2  VectorParamsAs1DForOutWhenUnconnected=off
  Out3 : Outport  Port=3  VectorParamsAs1DForOutWhenUnconnected=off
  Out4 : Outport  Port=4  VectorParamsAs1DForOutWhenUnconnected=off
  Out5 : Outport  Port=5  VectorParamsAs1DForOutWhenUnconnected=off
  Out6 : Outport  Port=6  VectorParamsAs1DForOutWhenUnconnected=off
  Out7 : Outport  Port=7  VectorParamsAs1DForOutWhenUnconnected=off
  Out8 : Outport  Port=8  VectorParamsAs1DForOutWhenUnconnected=off
  Out9 : Outport  Port=9  VectorParamsAs1DForOutWhenUnconnected=off
  wires:
  S-Function/9 -> Enabled Subsystem/8(In8)
  S-Function/4 -> Enabled Subsystem/3(In3)
  S-Function/5 -> Enabled Subsystem/4(In4)
  S-Function/8 -> Enabled Subsystem/7(In7)
  S-Function/7 -> Enabled Subsystem/6(In6)
  S-Function/6 -> Enabled Subsystem/5(In5)
  Enabled Subsystem/8(Out8) -> Out9/1
  Enabled Subsystem/7(Out7) -> Out8/1
  Enabled Subsystem/6(Out6) -> Out7/1
  Enabled Subsystem/5(Out5) -> Out6/1
  Enabled Subsystem/4(Out4) -> Out5/1
  Enabled Subsystem/3(Out3) -> Out4/1
  Enabled Subsystem/2(Out2) -> Out3/1
  Enabled Subsystem/1(Out1) -> Out2/1
  S-Function/3 -> Enabled Subsystem/2(In2)
  S-Function/2 -> Enabled Subsystem/1(In1)
  S-Function/1 -> Out1/1, Enabled Subsystem/Enable
  In1/1 -> S-Function/1

== system HANcoder_E407_TTA_Template_DS_V6/HANcoder STM32 Target - E407-STM32 algorithm/TTA CAN System/CAN2 Recieve1/RxID_CAN/Vote1_ID_CAN/CAN receive1 ==
  In1 : Inport
  Enabled Subsystem : Subsystem  TreatAsAtomicUnit=on
  S-Function : M-S-Function  FunctionName=sfcn_can_receive  Parameters=tsamp, canBus, outputNumber, dataType, byteOrder
  Out1 : Outport  VectorParamsAs1DForOutWhenUnconnected=off
  Out2 : Outport  Port=2  VectorParamsAs1DForOutWhenUnconnected=off
  Out3 : Outport  Port=3  VectorParamsAs1DForOutWhenUnconnected=off
  Out4 : Outport  Port=4  VectorParamsAs1DForOutWhenUnconnected=off
  Out5 : Outport  Port=5  VectorParamsAs1DForOutWhenUnconnected=off
  Out6 : Outport  Port=6  VectorParamsAs1DForOutWhenUnconnected=off
  Out7 : Outport  Port=7  VectorParamsAs1DForOutWhenUnconnected=off
  Out8 : Outport  Port=8  VectorParamsAs1DForOutWhenUnconnected=off
  Out9 : Outport  Port=9  VectorParamsAs1DForOutWhenUnconnected=off
  wires:
  In1/1 -> S-Function/1
  S-Function/1 -> Enabled Subsystem/Enable, Out1/1
  S-Function/2 -> Enabled Subsystem/1(In1)
  S-Function/3 -> Enabled Subsystem/2(In2)
  Enabled Subsystem/1(Out1) -> Out2/1
  Enabled Subsystem/2(Out2) -> Out3/1
  Enabled Subsystem/3(Out3) -> Out4/1
  Enabled Subsystem/4(Out4) -> Out5/1
  Enabled Subsystem/5(Out5) -> Out6/1
  Enabled Subsystem/6(Out6) -> Out7/1
  Enabled Subsystem/7(Out7) -> Out8/1
  Enabled Subsystem/8(Out8) -> Out9/1
  S-Function/6 -> Enabled Subsystem/5(In5)
  S-Function/7 -> Enabled Subsystem/6(In6)
  S-Function/8 -> Enabled Subsystem/7(In7)
  S-Function/5 -> Enabled Subsystem/4(In4)
  S-Function/4 -> Enabled Subsystem/3(In3)
  S-Function/9 -> Enabled Subsystem/8(In8)

== system HANcoder_E407_TTA_Template_DS_V6/HANcoder STM32 Target - E407-STM32 algorithm/TTA CAN System/CAN2 Recieve1/RxID_CAN/Vote2_ID_CAN/CAN receive1 ==
  In1 : Inport
  Enabled Subsystem : Subsystem  TreatAsAtomicUnit=on
  S-Function : M-S-Function  FunctionName=sfcn_can_receive  Parameters=tsamp, canBus, outputNumber, dataType, byteOrder
  Out1 : Outport  VectorParamsAs1DForOutWhenUnconnected=off
  Out2 : Outport  Port=2  VectorParamsAs1DForOutWhenUnconnected=off
  Out3 : Outport  Port=3  VectorParamsAs1DForOutWhenUnconnected=off
  Out4 : Outport  Port=4  VectorParamsAs1DForOutWhenUnconnected=off
  Out5 : Outport  Port=5  VectorParamsAs1DForOutWhenUnconnected=off
  Out6 : Outport  Port=6  VectorParamsAs1DForOutWhenUnconnected=off
  Out7 : Outport  Port=7  VectorParamsAs1DForOutWhenUnconnected=off
  Out8 : Outport  Port=8  VectorParamsAs1DForOutWhenUnconnected=off
  Out9 : Outport  Port=9  VectorParamsAs1DForOutWhenUnconnected=off
  wires:
  In1/1 -> S-Function/1
  S-Function/1 -> Enabled Subsystem/Enable, Out1/1
  S-Function/2 -> Enabled Subsystem/1(In1)
  S-Function/3 -> Enabled Subsystem/2(In2)
  Enabled Subsystem/1(Out1) -> Out2/1
  Enabled Subsystem/2(Out2) -> Out3/1
  Enabled Subsystem/3(Out3) -> Out4/1
  Enabled Subsystem/4(Out4) -> Out5/1
  Enabled Subsystem/5(Out5) -> Out6/1
  Enabled Subsystem/6(Out6) -> Out7/1
  Enabled Subsystem/7(Out7) -> Out8/1
  Enabled Subsystem/8(Out8) -> Out9/1
  S-Function/6 -> Enabled Subsystem/5(In5)
  S-Function/7 -> Enabled Subsystem/6(In6)
  S-Function/8 -> Enabled Subsystem/7(In7)
  S-Function/5 -> Enabled Subsystem/4(In4)
  S-Function/4 -> Enabled Subsystem/3(In3)
  S-Function/9 -> Enabled Subsystem/8(In8)

== system HANcoder_E407_TTA_Template_DS_V6/HANcoder STM32 Target - E407-STM32 algorithm/TTA CAN System/CAN2 Recieve1/RxID_CAN/Vote3_ID_CAN/CAN receive1 ==
  In1 : Inport
  Enabled Subsystem : Subsystem  TreatAsAtomicUnit=on
  S-Function : M-S-Function  FunctionName=sfcn_can_receive  Parameters=tsamp, canBus, outputNumber, dataType, byteOrder
  Out1 : Outport  VectorParamsAs1DForOutWhenUnconnected=off
  Out2 : Outport  Port=2  VectorParamsAs1DForOutWhenUnconnected=off
  Out3 : Outport  Port=3  VectorParamsAs1DForOutWhenUnconnected=off
  Out4 : Outport  Port=4  VectorParamsAs1DForOutWhenUnconnected=off
  Out5 : Outport  Port=5  VectorParamsAs1DForOutWhenUnconnected=off
  Out6 : Outport  Port=6  VectorParamsAs1DForOutWhenUnconnected=off
  Out7 : Outport  Port=7  VectorParamsAs1DForOutWhenUnconnected=off
  Out8 : Outport  Port=8  VectorParamsAs1DForOutWhenUnconnected=off
  Out9 : Outport  Port=9  VectorParamsAs1DForOutWhenUnconnected=off
  wires:
  In1/1 -> S-Function/1
  S-Function/1 -> Enabled Subsystem/Enable, Out1/1
  S-Function/2 -> Enabled Subsystem/1(In1)
  S-Function/3 -> Enabled Subsystem/2(In2)
  Enabled Subsystem/1(Out1) -> Out2/1
  Enabled Subsystem/2(Out2) -> Out3/1
  Enabled Subsystem/3(Out3) -> Out4/1
  Enabled Subsystem/4(Out4) -> Out5/1
  Enabled Subsystem/5(Out5) -> Out6/1
  Enabled Subsystem/6(Out6) -> Out7/1
  Enabled Subsystem/7(Out7) -> Out8/1
  Enabled Subsystem/8(Out8) -> Out9/1
  S-Function/6 -> Enabled Subsystem/5(In5)
  S-Function/7 -> Enabled Subsystem/6(In6)
  S-Function/8 -> Enabled Subsystem/7(In7)
  S-Function/5 -> Enabled Subsystem/4(In4)
  S-Function/4 -> Enabled Subsystem/3(In3)
  S-Function/9 -> Enabled Subsystem/8(In8)

== system HANcoder_E407_TTA_Template_DS_V6/HANcoder STM32 Target - E407-STM32 algorithm/TTA CAN System/TTA System/Initialization/RoleID and Global Time init/Global Time Initialization Master ==
  note: Global Time Initialization
  Enable : EnablePort
  Board nr1 : Constant
  Cast : DataTypeConversion  OutDataTypeStr=uint16  SaturateOnIntegerOverflow=off  RndMeth=Floor
  Cast1 : DataTypeConversion  OutDataTypeStr=uint8  SaturateOnIntegerOverflow=off  RndMeth=Floor
  Data Store Write : DataStoreWrite  DataStoreName=Local_Ticks  IndexOptions=Index vector (dialog)  Indices=1  OutputSizes=1
  Data Store Write1 : DataStoreWrite  DataStoreName=basic_cycle_count  IndexOptions=Index vector (dialog)  Indices=1  OutputSizes=1
  Data Store Write3 : DataStoreWrite  DataStoreName=Master_ID  IndexOptions=Index vector (dialog)  Indices=1  OutputSizes=1
  Start : Constant  Value=0
  wires:
  Board nr1/1 -> Data Store Write3/1
  Start/1 -> Cast1/1, Cast/1
  Cast/1 -> Data Store Write/1
  Cast1/1 -> Data Store Write1/1

== system HANcoder_E407_TTA_Template_DS_V6/HANcoder STM32 Target - E407-STM32 algorithm/TTA CAN System/TTA System/Initialization/RoleID and Global Time init/Global Time Initialization Slave ==
  note: Sync has already been received, so we skip
      | the first comp tasks related to Update LT.
  note: Global Time Initialization
  note: Estimation of the Local Time when the message was sent
  Enable : EnablePort
  Bus Selector : BusSelector  OutputSignals=Buffer_1,Buffer_2,Buffer_3,Buffer_4,Buffer_5,Buffer_6,Buffer_7,Buffer_8
  Cast : DataTypeConversion  OutDataTypeStr=uint16  SaturateOnIntegerOverflow=off  RndMeth=Floor
  Cast1 : DataTypeConversion  OutDataTypeStr=double  SaturateOnIntegerOverflow=off  RndMeth=Floor
  Constant : Constant
  Constant1 : Constant  Value=COMM_Phase1
  Constant2 : Constant  Value=COMM_Phase2
  Constant3 : Constant  Value=TM_COMM_Sync
  Data Store Read : DataStoreRead  DataStoreName=New_Msg_Ready_CAN1  IndexOptions=Index vector (dialog)  Indices=1  OutputSizes=1
  Data Store Read1 : DataStoreRead  DataStoreName=Msg_Rx_CAN1  IndexOptions=Index vector (dialog)  Indices=1  OutputSizes=1
  Data Store Read2 : DataStoreRead  DataStoreName=Msg_Rx_CAN2  IndexOptions=Index vector (dialog)  Indices=1  OutputSizes=1
  Data Store Write1 : DataStoreWrite  DataStoreName=Local_Ticks  IndexOptions=Index vector (dialog)  Indices=1  OutputSizes=1
  Data Store Write2 : DataStoreWrite  DataStoreName=basic_cycle_count  IndexOptions=Index vector (dialog)  Indices=1  OutputSizes=1
  Data Store Write3 : DataStoreWrite  DataStoreName=Master_ID  IndexOptions=Index vector (dialog)  Indices=1  OutputSizes=1
  Data Store Write4 : DataStoreWrite  Priority=10  DataStoreName=BC0_Sync_processed  IndexOptions=Index vector (dialog)  Indices=1  OutputSizes=1
  Equal : RelationalOperator  Operator===  OutDataTypeStr=boolean  RndMeth=Simplest  InputSameDT=off
  Multiply : Product
  Multiply1 : Product
  "SET1 " : Constant  Priority=9  OutDataTypeStr=boolean
  Sum : Sum  Inputs=+++
  Sum1 : Sum  Inputs=+++
  Switch : Switch  Criteria=u2 > Threshold  SaturateOnIntegerOverflow=off  InputSameDT=off
  Switch1 : Switch  Criteria=u2 > Threshold  SaturateOnIntegerOverflow=off  InputSameDT=off
  Terminator{1..7} (7 alike) : Terminator
  delay_estimation_1 : Constant  Value=comm_delay_estimation1
  delay_estimation_2 : Constant  Value=comm_delay_estimation2
  msg_decoding : Subsystem
  wires:
  Data Store Read/1 -> Equal/1
  Constant/1 -> Equal/2
  Bus Selector/8 -> Terminator7/1  "<Buffer_8>"
  Bus Selector/7 -> Terminator6/1  "<Buffer_7>"
  Switch/1 -> Bus Selector/1
  Bus Selector/1 -> msg_decoding/1(Msg_Temporal_Data)  "<Buffer_1>"
  Equal/1 -> Switch/2, [Rx_CAN1]
  Data Store Read1/1 -> Switch/1
  Data Store Read2/1 -> Switch/3
  "SET1 "/1 -> Data Store Write4/1
  msg_decoding/1(basic_cycle) -> Data Store Write2/1  "Rx_init_bc"
  msg_decoding/3(board_id) -> Cast1/1  "Rx_init_id"
  Constant3/1 -> Sum/2, Sum1/2
  Constant2/1 -> Multiply1/1
  Constant1/1 -> Multiply/1
  delay_estimation_2/1 -> Sum1/3
  Sum/1 -> Switch1/1
  msg_decoding/2(msg_count) -> Multiply/2, Multiply1/2  "Rx_init_mc"
  Multiply/1 -> Sum/1
  Multiply1/1 -> Sum1/1
  Sum1/1 -> Switch1/3
  delay_estimation_1/1 -> Sum/3
  [Rx_CAN1] -> Switch1/2
  Switch1/1 -> Cast/1
  Cast/1 -> Data Store Write1/1  "Rx_init_LT"
  Cast1/1 -> Data Store Write3/1
  Bus Selector/2 -> Terminator5/1  "<Buffer_2>"
  Bus Selector/3 -> Terminator2/1  "<Buffer_3>"
  Bus Selector/4 -> Terminator3/1  "<Buffer_4>"
  Bus Selector/5 -> Terminator4/1  "<Buffer_5>"
  Bus Selector/6 -> Terminator1/1  "<Buffer_6>"

== system HANcoder_E407_TTA_Template_DS_V6/HANcoder STM32 Target - E407-STM32 algorithm/TTA CAN System/TTA System/Matrix Cycle Manager/Controller Matrix Cycle/Matrix_Cycle_Observation_DEBUG ==
  Data Store Read : DataStoreRead  DataStoreName=Master_ID  IndexOptions=Index vector (dialog)  Indices=1  OutputSizes=1
  Data Store Read1 : DataStoreRead  DataStoreName=Role_ID  IndexOptions=Index vector (dialog)  Indices=1  OutputSizes=1
  Data Store Read10 : DataStoreRead  DataStoreName=BC1_Sync_processed  IndexOptions=Index vector (dialog)  Indices=1  OutputSizes=1
  Data Store Read11 : DataStoreRead  DataStoreName=Sync_bc0_missed_counter  IndexOptions=Index vector (dialog)  Indices=1  OutputSizes=1
  Data Store Read12 : DataStoreRead  DataStoreName=Sync_bc1_missed_counter  IndexOptions=Index vector (dialog)  Indices=1  OutputSizes=1
  Data Store Read2 : DataStoreRead  DataStoreName=BC0_Sync_processed  IndexOptions=Index vector (dialog)  Indices=1  OutputSizes=1
  Data Store Read3 : DataStoreRead  DataStoreName=Votes_count  DataStoreElements=Votes_count.First_Board#Votes_count.Second_Board#Votes_count.Third_Board  IndexOptions=Index vector (dialog)  Indices=1  OutputSizes=1
  Data Store Read4 : DataStoreRead  DataStoreName=Board1_error_counter  IndexOptions=Index vector (dialog)  Indices=1  OutputSizes=1
  Data Store Read5 : DataStoreRead  DataStoreName=Board2_error_counter  IndexOptions=Index vector (dialog)  Indices=1  OutputSizes=1
  Data Store Read6 : DataStoreRead  DataStoreName=Board3_error_counter  IndexOptions=Index vector (dialog)  Indices=1  OutputSizes=1
  Data Store Read7 : DataStoreRead  DataStoreName=BC0_Vote1_processed  IndexOptions=Index vector (dialog)  Indices=1  OutputSizes=1
  Data Store Read8 : DataStoreRead  DataStoreName=BC0_Vote2_processed  IndexOptions=Index vector (dialog)  Indices=1  OutputSizes=1
  Data Store Read9 : DataStoreRead  DataStoreName=BC0_Vote3_processed  IndexOptions=Index vector (dialog)  Indices=1  OutputSizes=1
  Terminator{,1..12,14..15} (15 alike) : Terminator
  wires:
  Data Store Read/1 -> Terminator1/1  "Master_ID_s"
  Data Store Read3/1 -> Terminator5/1  "votes_Board_1_DEBUG"
  Data Store Read3/2 -> Terminator6/1  "votes_Board_2_DEBUG"
  Data Store Read3/3 -> Terminator7/1  "votes_Board_3_DEBUG"
  Data Store Read4/1 -> Terminator8/1  "Board_1_error_counter_s"
  Data Store Read5/1 -> Terminator9/1  "Board_2_error_counter_s"
  Data Store Read6/1 -> Terminator10/1  "Board_3_error_counter_s"
  Data Store Read2/1 -> Terminator2/1  "BC0_sync_processed_s"
  Data Store Read7/1 -> Terminator3/1  "BC0_vote1_processed_s"
  Data Store Read8/1 -> Terminator4/1  "BC0_vote2_processed_s"
  Data Store Read9/1 -> Terminator11/1  "BC0_vote3_processed_s"
  Data Store Read10/1 -> Terminator12/1  "BC1_sync_processed_s"
  Data Store Read1/1 -> Terminator/1  "Role_ID_s"
  Data Store Read11/1 -> Terminator14/1  "sync_bc0_miss_counter_s"
  Data Store Read12/1 -> Terminator15/1  "sync_bc1_miss_counter_s"
